simulink model "simulation_model"  (R2022a)
settings: Solver=VariableStepAuto  StartTime=0.0  StopTime=inf  FixedStep=0.02  MaxStep=0.1  RelTol=1e-3
values from neighbouring files (symbols this model uses):
  psi0 = atan(yc/xc)    [close_example.m]    (also in example_m.m)
  xc = coordinate(1)    [close_example.m]    (also in example_m.m)
  yc = coordinate(2)    [close_example.m]    (also in example_m.m)
undefined symbols (not defined in the file or in its folder): fuel_rate, gamma_pb, Pose, sigbuilder_block
libraries: simulink_extras x4, robotlib x3, simulink x1
(part 2 of 3)

== matlab function simulation_model/Rocket control model/proportional navigation ==
  data: t input; xc input; K_w output; yc input; x input; y input; beta input; alfa input; psi input; theta input; z input; K_k output
%% function which calculates control commands for fins in proportional navigation
% 
% Inputs:
% t - time of flight [s] 
% xc, yc - coordinates of the target 
% x, y, z - coordinates of the rocket
% alfa - angle of attack [rad]
% beta -  angle of sideslip [rad]
% theta - pitch angle [rad]
% psi - yaw angle [rad]
%
% Outputs:
% K_w - command control of fins in axis Z
% K_k - command control of fins in axis Y

function [K_w, K_k] = fcn(t, xc, yc, x, y, beta, alfa, psi, theta, z)

%guidance angles
epsilon_theta = atan(z/sqrt((xc-x)^2 + (yc-y)^2));
epsilon_psi = atan((yc-y)/(xc-x));

%velocity vector angles
gamma = theta - alfa;
gamma2 = psi - beta;

%guidance error angles
u1 = epsilon_theta - (gamma);
u2 = epsilon_psi - (gamma2);

% fins deflection limit in axis Z
kat = 7;

%command control of fins in axis Z
if u1 < 0 && t > 100 && z > -8000
    K_w = -100*pi*u1;
    if abs(K_w) > kat
        K_w = deg2rad(kat);
    else
        K_w = deg2rad(K_w);
    end
   
     
elseif u1 > 0 && t > 100 && z > -8000
    K_w = 100*pi*u1;
    if abs(K_w) > kat
        K_w = deg2rad(-kat);
    else
        K_w = deg2rad(K_w);
    end
   
    
else
    K_w = 0;
end

% fins deflection limit in axis Y
kat = 0; 

%command control of fins in axis Y
if u2 < 0 && t > 100 && z > -8000
    K_k = -50*pi*u2.^2;
    if abs(K_k) > kat
        K_k = deg2rad(-kat);
    else
        K_k = deg2rad(K_w);
    end
    
     
elseif u2 > 0 && t > 100 && z > -31000
    K_k = 50*pi*u2.^2;
    if abs(K_k) > kat
        K_k = deg2rad(kat);
    else
        K_k = deg2rad(K_w);
    end
    
else
    K_k = 0;
end

== matlab function simulation_model/Rocket control model/programmable aerodynamic control ==
  data: gamma_p input; psi_p input; z input; z_dot input; theta input; psi input; alfa input; beta input; t input; K_w output; K_k output
%% function which calculates control commands for fins
% 
% Inputs:
%gamma_p - programmable pith angle [rad]
% psi_p - programmable yaw angle [rad]
% z - altitude [m]
% z_dot - the derivative of altitude [m/s]
% theta - pitch angle [rad]
% psi - yaw angle [rad]
% alfa - angle of attack [rad]
% beta -  angle of sideslip [rad]
% t - time of flight [s]
%
% Outputs:
% K_w - command control of fins in axis Z
% K_k - command control of fins in axis Y


function [K_w, K_k] = fcn(gamma_p, psi_p, z, z_dot, theta, psi, alfa, beta, t)

%velocity vector angles
gamma = theta - alfa;
gamma2 = psi - beta;

%midcourse phase
if z_dot > 0 && z < -25000  

    %guidance error angles
    u1 = gamma_p - (gamma);
    u2 = psi_p - (gamma2);
    
    % fins deflection limit
    kat = 0;
    
    %command control of fins in axis Z
    if u1 < 0 
        K_w = -100*u1;
        if abs(K_w) > kat
            K_w = deg2rad(kat);
        else
            K_w = deg2rad(K_w);
        end
         
    elseif u1 > 0 
        K_w = -100*u1;
        if abs(K_w) > kat
            K_w = deg2rad(-kat);
        else
            K_w = deg2rad(K_w);
        end
    else 
        K_w = 0;
    end
    
    %command control of fins in axis Y
    if u2 < 0 
        K_k = -0.001*u2;
        if abs(K_k) > kat
            K_k = deg2rad(kat);
        else
            K_k = deg2rad(K_k);
        end
         
    elseif u2 > 0 
        K_k = -0.001*u2;
        if abs(K_k) > kat
            K_k = deg2rad(-kat);
        else
            K_k = deg2rad(K_k);
        end
    else 
        K_k = 0;
    end


% terminal phase
elseif t > 200 && z > -20000 && z < -12000
    
    % programmable angle
    gamma_p = deg2rad(-90);

    % fins deflection limit in axis Z
    kat = 10;
    
    %guidance error angles
    u1 = gamma_p - (gamma);
    u2 = psi_p - (gamma2);
    
    %command control of fins in axis Z
    if u1 < 0
        K_w = 38*pi*u1.^2;
        if abs(K_w) > kat
            K_w = deg2rad(kat);
        else
            K_w = deg2rad(K_w);
        end
         
    elseif u1 > 0
        K_w = -2*pi*u1;
        if abs(K_w) > kat
            K_w = deg2rad(-kat);
        else
            K_w = deg2rad(K_w);
        end
    else
        K_w = 0;
    end

    %command control of fins in axis Y
    if u2 < 0 
        K_k = -0.0001*u2;
        if abs(K_k) > kat
            K_k = deg2rad(kat);
        else
            K_k = deg2rad(K_k);
        end
         
    elseif u2 > 0 
        K_k = -0.0001*u2;
        if abs(K_k) > kat
            K_k = deg2rad(-kat);
        else
            K_k = deg2rad(K_k);
        end
    else 
        K_k = 0;
    end

else
    K_w = 0;
    K_k = 0;
end

== matlab function simulation_model/Parameters of rocket 9M723 and atmosphere model/Atmosphere model ISO 2533 ==
  data: h input; g output; a output; rho output; p output
%% function which calculates parameters of Atmosphere
% 
% Inputs:
% h - alltitude of rocket [m];
%
% Outputs:
% g - gravitational acceleration [m/s^2]
% a - speed of sound [m/s]
% rho - air density [kg/m^3]
% p - pressure [Pa]

function [g, a, rho, p] = fcn(h)

h = abs(h);
R_o = 287.05287; %proper gas constant
g_n = 9.80665; %exemplary gravitational acceleration [m/s^2]
R_z = 6356766;%the nominal radius of the Earth [m]
H = R_z*h/(R_z+h); %geopotential alltitude
H = H/1000; % [m] -> [km]

%gravitational acceleration
g = g_n.*(R_z./(R_z+h)).^2; 

%temperature 
if H < 0
        T = 301.15 - 6.5.*(H+2);
    elseif H >= 0 && H < 11
        T = 288.15 - 6.5.*(H-0);
    elseif H >= 11 && H < 20
        T = 216.65 + 0.*(H-11);
    elseif H >= 20 && H < 32
        T = 216.65 + 1.*(H-20);
    elseif H >= 32 && H < 47
        T = 228.65 + 2.8.*(H-32);
    elseif H >= 47 && H < 51
        T = 270.65 + 0.*(H-47);
    elseif H >= 51 && H < 71
        T = 270.65 - 2.8.*(H-51);
    elseif H >= 71 && H < 80
        T = 214.65 - 2.*(H-71);
    else
        T = 196.65;
end

% speed of sound
a = 20.046796.*sqrt(T);

%pressure
g_n = g_n*1e-3; %[m] -> [km]
R_o = R_o*1e-6;

if H < 0
        p = 127783*(1-6.5/301.15*(H+2))^(-g_n/(-6.5*R_o));
    elseif H >= 0 && H < 11
        p = 101325*(1-6.5/288.15*(H-0))^(-g_n/(-6.5*R_o));
    elseif H >= 11 && H < 20
        p = 22632*exp(-g_n/R_o/T*(H-11));
    elseif H >= 20 && H < 32
        p = 5474.9*(1+1/216.65*(H-20))^(-g_n/(1*R_o));
    elseif H >= 32 && H < 47
        p = 868.02*(1+2.8/228.65*(H-32))^(-g_n/(2.8*R_o));
    elseif H >= 47 && H < 51
        p = 110.91*exp(-g_n/R_o/T*(H-47));
    elseif H >= 51 && H < 71
        p = 66.939*(1-2.8/270.65*(H-51))^(-g_n/(-2.8*R_o));
    elseif H >= 71 && H < 80
        p = 3.9564*(1-2/214.65*(H-71))^(-g_n/(-2*R_o));
    else
        p = 0.3734;
end

% air density
R_o = R_o*1e+6; %[km] -> [m]
rho = p./R_o./T;

== matlab function simulation_model/Parameters of rocket 9M723 and atmosphere model/Mass-inertia characteristics 9M723 ==
  data: m output; x_sm output; I_x output; I output; fuel input
%% function which calculates parameters mass-inertia characteristics determined with data from Autocad
% 
% Inputs:
% fuel - percent of rocket fuel[%];
%
% Outputs:
% m - mass of rocket [kg]
% x_sm - center of gravity [m]
% I_x - moment of inertia Ix [kg*m^2]
% I - moments of inertia Iy and Iz [kg*m^2]

function [m, x_sm, I_x, I] = fcn(fuel)

% percent of rocket fuel
fuel_w = [0 5 10 15 20 25 30 35 40 45 50 55 60 65 70 75 80 85 90 95 100];

% calculate mass of the rocket
% mass of rocket with 100% fuel - 4615 kg
% mass of rocket fuel - 2920 kg
p_m = polyfit([0 100],[4615-2920  4615],1);
masa_obl = p_m(1).*fuel_w + p_m(2); 

% solid volume
V = [1312001487.1908  
    1391194465.7760 
    1470387444.3611 
    1549580422.9463 
    1628773401.5315 
    1707966380.1166 
    1787159358.7018
    1866352337.2870 
    1945545315.8721
    2024738294.4573
    2103931273.0425
    2183124251.6276  
    2262317230.2128
    2341510208.7980 
    2420703187.3831
    2499896165.9683
    2579089144.5535
    2658282123.1386 
    2737475101.7238
    2816668080.3090
    2895861058.8942 ];

% Center of Gravity
CG = [2810.7476 
    2875.9405 
    2941.2203 
    3006.5737 
    3071.9900 
    3137.4604 
    3202.9778
    3268.5361
    3334.1304
    3399.7564
    3465.4105
    3531.0898
    3596.7915 
    3662.5134 
    3728.2535 
    3794.0100 
    3859.7815
    3925.5666
    3991.3642
    4057.1731
    4122.9925 ];

% moments of inertia [I_x I_y I_z]
M_bezw = [1.0009E+14 2661071015412923 2661071018604918
    1.0765E+14 2762923872394703 2762923875586698 
    1.1522E+14 2876895198158699 2876895201350695 
    1.2278E+14 3003675169911807 3003675173103802 
    1.3034E+14 3143953916633058 3143953919825051 
    1.3790E+14 3298421530254443 3298421533446437 
    1.4546E+14 3467768073869122 3467768077061116 
    1.5302E+14 3652683587849863 3652683591041859 
    1.6059E+14 3853858094473163 3853858097665158 
    1.6815E+14 4071981601458265 4071981604650260 
    1.7571E+14 4307744104706791 4307744107898786 
    1.8327E+14 4561835590446237 4561835593638231 
    1.9083E+14 4834946036923169 4834946040115163 
    1.9839E+14 5127765415752858 5127765418944854 
    2.0596E+14 5440983693004008 5440983696196001 
    2.1352E+14 5775290830077207 5775290833269201 
    2.2108E+14 6131376784421738 6131376787613735 
    2.2864E+14 6509931510124066 6509931513316063 
    2.3620E+14 6911644958394299 6911644961586294 
    2.4377E+14 7337207077970520 7337207081162515 
    2.5133E+14 7787307815456737 7787307818648729];

% calculate Autocad factor which provide the ability to calculate real parameters
WSP = masa_obl'./V./1e6;

% calculate real moments of inertia
M_bezw = M_bezw.*WSP;

% calculate mass-inertia characteristics
if fuel >= 100
    m = masa_obl(end);
    x_sm = CG(end)/1000;
    I_x = M_bezw(end,1);
    I = M_bezw(end,2);
elseif fuel <= 0
    m = masa_obl(1);
    x_sm = CG(1)/1000;
    I_x = M_bezw(1,1);
    I = M_bezw(1,2);
else
    p = polyfit(fuel_w,masa_obl,2);
    m = polyval(p,fuel);

    p = polyfit(fuel_w,CG,2);
    x_sm = polyval(p,fuel)/1000;

    p = polyfit(fuel_w,M_bezw(:,1),3);
    I_x = polyval(p,fuel);

    p = polyfit(fuel_w,M_bezw(:,2),3);
    I = polyval(p,fuel);
end
